simulink model "TV_2017old"  (R2016a)
settings: Solver=FixedStepAuto  StartTime=0.0  StopTime=inf  FixedStep=0.001  RelTol=1e-3
PreLoadFcn:
  | TV_2017_parameters
values from neighbouring files (symbols this model uses):
  battery_voltage = single(530)    [HIL_parameters.m]    (also in HIL_parameters_2018.m; TV_2017_parameters.m; TV_2017_parameters_VD.m)
  car_params = Simulink_Car_params    [HIL_parameters.m]    (also in HIL_parameters_2018.m; TV_2017_parameters.m; TV_2017_parameters_VD.m)
  i_Diff = 16    [HIL_parameters.m]    (also in HIL_parameters_2018.m; TV_2017_parameters.m)
  Kp = 1    [HIL_parameters.m]    (also in HIL_parameters_2018.m; TV_2017_parameters.m; TV_2017_parameters_VD.m)
  motor_data = struct    [HIL_parameters.m]    (also in HIL_parameters_2018.m; TV_2017_parameters.m)
  powerLimitControl = Simulink_el    [HIL_parameters.m]    (also in HIL_parameters_2018.m; TV_2017_parameters.m; TV_2017_parameters_VD.m)
  settings = Simulink_Settings    [HIL_parameters.m]    (also in HIL_parameters_2018.m; TV_2017_parameters.m; TV_2017_parameters_VD.m)
  SpdC_BCC = 0    [HIL_parameters.m]    (also in HIL_parameters_2018.m; TV_2017_parameters.m; TV_2017_parameters_VD.m)
  Speed_Neg_sat = -21    [HIL_parameters.m]    (also in HIL_parameters_2018.m; TV_2017_parameters.m; TV_2017_parameters_VD.m)
  Speed_Pos_sat = 21    [HIL_parameters.m]    (also in HIL_parameters_2018.m; TV_2017_parameters.m; TV_2017_parameters_VD.m)
  SteeringAngleFL = [-23.80 -22.65 -21.50 -20.34 -19.18 -18.03 -16.86 -15.70 -14.53 -13.35 -12.18 -10.99 -9.80 -8.61 -7.40 -6.19 -4.97 -3.75 -2.51 -1.26 0 1.27 2.56 3.85 5.17 6.50 7.84 9.21 10.59 12.00 13.42 14.88 16.36 17.87 19.41 20.99 22.61 24.26 25.97 27.73 29.54]    [CarSetupAnalysis2018.m]    (also in HIL_parameters_2018.m; TV_2017_parameters.m; TV_2017_parameters_VD.m = [-24.129 -22.950 -21.772 -20.593 -19.413 -18.232 -17.050 -15)
  SteeringAngleFR = [-29.54 -27.73 -25.97 -24.26 -22.61 -20.99 -19.41 -17.87 -16.36 -14.88 -13.42 -12.00 -10.59 -9.21 -7.84 -6.50 -5.17 -3.85 -2.56 -1.27 0 1.26 2.51 3.75 4.97 6.19 7.40 8.61 9.80 10.99 12.18 13.35 14.53 15.70 16.86 18.03 19.18 20.34 21.50 22.65 23.80]    [CarSetupAnalysis2018.m]    (also in HIL_parameters_2018.m; TV_2017_parameters.m; TV_2017_parameters_VD.m = [-29.3050 -27.5340 -25.8140 -24.1410 -22.5110 -20.9180 -19.3)
  SteeringWhAngle = [-105 -99.75 -94.5 -89.25 -84 -78.75 -73.5 -68.25 -63 -57.75 -52.5 -47.25 -42 -36.75 -31.5 -26.25 -21.0 -15.75 -10.5 -5.25 0.0 5.25 10.50 15.75 21.00 26.25 31.50 36.75 42.00 47.25 52.50 57.75  63.00 68.25 73.50 78.75 84.00 89.25 94.50 99.75 105.00]    [TV_2017_parameters_VD.m]
  Tn_n = 0    [HIL_parameters.m]    (also in HIL_parameters_2018.m; TV_2017_parameters.m; TV_2017_parameters_VD.m)
  tractionControl = Simulink_tc    [HIL_parameters.m]    (also in HIL_parameters_2018.m; IterativeTractionControlTuning.m; TV_2017_parameters.m; TV_2017_parameters_VD.m)
  yawRateControl = Simulink_yawRate    [HIL_parameters.m]    (also in HIL_parameters_2018.m; TV_2017_parameters.m; TV_2017_parameters_VD.m)
undefined symbols (not defined in the file or in its folder): DiscIntNeverNeededParam, magnitude, speedEstimation, TC_Decr_Gas, TC_Derivative, TC_Incr_Gas, TC_On, TC_Relay_Off, TC_Relay_On
libraries: CarMaker4SL x274, simulink_extras x45, simulink x37, dspfdesign x2
(part 11 of 14)

== matlab function TV_2017old/CarMaker/Control_System /TA 2017/TorqueAllocation ==
  data: Mz_ref input; Ti_lim output Bus: Ti_lim; T_req input; states input; maxMotorTorque input; friction_limit_torques input; settings parameter; car_params parameter; pow_red output; yawRateControl parameter; powerLimitControl parameter; Mz_error output; Mz_allocated output; overiterate output
function [Ti_lim, pow_red,Mz_error, Mz_allocated,overiterate] = torqueAllocation(Mz_ref, T_req, states, maxMotorTorque, friction_limit_torques, settings, car_params, yawRateControl, powerLimitControl)
saturated_constraints = int8([0 0 0 0]);
Mz_error = single(0);
Mz_allocated = single(0);
pow_red = int8([0 0 0 0]);
overiterate = int8(0);




switch settings.TV_Method
    case 1 
        [Ti_lim, pow_red,Mz_error, Mz_allocated] = TA_17(Mz_ref, T_req, states, maxMotorTorque,friction_limit_torques, settings, car_params, yawRateControl, powerLimitControl);    
    case 2
        [Ti_lim,Ti_max,Mz_error, Mz_allocated] = TA_16(T_req,states,maxMotorTorque,settings, car_params, Mz_ref,yawRateControl);   
    case 3
        [Ti_lim,Ti_max,Mz_error, Mz_allocated] = TA_16(T_req,states,maxMotorTorque,settings, car_params, Mz_ref,yawRateControl);
    case 4
        [Ti_lim,Ti_max,Mz_error, Mz_allocated] = TA_16(T_req,states,maxMotorTorque,settings, car_params, Mz_ref,yawRateControl);
    otherwise
        Ti_lim_struct.FL =  single(0); Ti_lim_struct.FR =  single(0); Ti_lim_struct.RL = single(0); Ti_lim_struct.RR =  single(0);
        Ti_lim = Ti_lim_struct;
      
end





end
%{
function [Ti_lim, saturated_constraints,Mz_error, Mz_allocated] = TA_17(Mz_ref, T_req, states, maxMotorTorque,friction_limit_torques, settings, car_params, yawRateControl, powerLimitControl)

%-----variables
error = 0;
pow_red = 0;
max_matrix_dimention = 17;
Ti_max = [0 0 0 0];
Mz_allocated = single(0);
saturated_constraints = int8([0 0 0 0]);
pow_lim_en = powerLimitControl.enable;

% ------- STATES -------------
r = states.r;
negative_torque_limit = yawRateControl.negative_torque_limit;

%---------- PARAMETERS -------
TV_method = settings.TV_Method;
% motor torque limits  
max_motor_torque = single(settings.max_motor_torque);  % absolute limit
negative_torque_limit = yawRateControl.negative_torque_limit;   % max negative DYC torque while accelerating
max_motor_brake_torque = settings.max_motor_brake_torque;   % max brake torque (decelerating)

mu = settings.mu;
lf = car_params.l_f;
lr = car_params.l_r;
tf = car_params.t_f;
tr = car_params.t_r;
arm_f = sqrt(tf^2 + lf^2);
GR = car_params.GR;
r_eff = car_params.r_eff;
R = [r_eff, r_eff, r_eff, r_eff]; % todo -> account for load
delta = states.wheel_angle;
delta_FL = delta;   % fix for later  ->individual steer angles
delta_FR = delta;
T_abs = abs(T_req); 
Mz_ref_scaled = single(Mz_ref * single(yawRateControl.enable));
Mz_min = -yawRateControl.max_moment;
Mz_max = yawRateControl.max_moment;
pow_lim         = powerLimitControl.positive_power_limit; %= single(75000); % Positive effect limit
neg_pow_lim     = powerLimitControl.negative_power_limit;
V_x = states.V_x;



rads_FL = max(10,abs(states.RPM_FL))*2*pi/60  ;
rads_FR = max(10,abs(states.RPM_FR))*2*pi/60  ;
rads_RL = max(10,abs(states.RPM_RL))*2*pi/60  ;
rads_RR = max(10,abs(states.RPM_RR))*2*pi/60  ;

RPM_FL = single(max(500,states.RPM_FL));
RPM_FR = single(max(500,states.RPM_FR));
RPM_RL = single(max(500,states.RPM_RL));
RPM_RR = single(max(500,states.RPM_RR));

mmt_FL = min(max_motor_torque, max(0.1, maxMotorTorque.mmt_FL));  % indivudual max torques
mmt_FR = min(max_motor_torque, max(0.1, maxMotorTorque.mmt_FR)); 
mmt_RL = min(max_motor_torque, max(0.1, maxMotorTorque.mmt_RL)); 
mmt_RR = min(max_motor_torque, max(0.1, maxMotorTorque.mmt_RR));

minmt_FL = min([mmt_FL max_motor_brake_torque]);  % indivudual min torques
minmt_FR = min([mmt_FR max_motor_brake_torque]);
minmt_RL = min([mmt_RL max_motor_brake_torque]);
minmt_RR = min([mmt_RR max_motor_brake_torque]);

max_neg_corr_torque_FL = min([minmt_FL negative_torque_limit]);  % indivudual min torques as corrective moment during acceleration
max_neg_corr_torque_FR = min([minmt_FR negative_torque_limit]); 
max_neg_corr_torque_RL = min([minmt_RL negative_torque_limit]);
max_neg_corr_torque_RR = min([minmt_RR negative_torque_limit]);

%***************************************************


%***************************************************
motor_eff_table = single(100*reshape([0.6437000036239624,0.5799999833106995,0.44999998807907104,0.3499999940395355,0.28999999165534973,0.23999999463558197,0.20000000298023224,0.17000000178813934,0.14000000059604645,0.12999999523162842,0.10999999940395355,0.7099999785423279,0.699999988079071,0.6100000143051148,0.5099999904632568,0.4399999976158142,0.3799999952316284,0.33000001311302185,0.28999999165534973,0.25,0.2199999988079071,0.20000000298023224,0.7300000190734863,0.7699999809265137,0.7300000190734863,0.6700000166893005,0.6100000143051148,0.550000011920929,0.5,0.44999998807907104,0.4000000059604645,0.36000001430511475,0.33000001311302185,0.7400000095367432,0.800000011920929,0.7900000214576721,0.7400000095367432,0.6899999976158142,0.6399999856948853,0.5899999737739563,0.5400000214576721,0.5,0.46000000834465027,0.41999998688697815,0.75,0.8199999928474426,0.8199999928474426,0.7799999713897705,0.7400000095367432,0.699999988079071,0.6600000262260437,0.6100000143051148,0.5699999928474426,0.5299999713897705,0.49000000953674316,0.7599999904632568,0.8399999737739563,0.8500000238418579,0.8299999833106995,0.800000011920929,0.7699999809265137,0.7400000095367432,0.699999988079071,0.6600000262260437,0.6200000047683716,0.5899999737739563,0.7699999809265137,0.8500000238418579,0.8799999952316284,0.8700000047683716,0.8600000143051148,0.8399999737739563,0.8100000023841858,0.7799999713897705,0.7599999904632568,0.7200000286102295,0.699999988079071,0.7699999809265137,0.8500000238418579,0.8899999856948853,0.8799999952316284,0.8700000047683716,0.8500000238418579,0.8299999833106995,0.8100000023841858,0.7799999713897705,0.7599999904632568,0.7300000190734863,0.7699999809265137,0.8600000143051148,0.8999999761581421,0.8999999761581421,0.8899999856948853,0.8700000047683716,0.8500000238418579,0.8299999833106995,0.8100000023841858,0.7900000214576721,0.6700000166893005,0.7799999713897705,0.8600000143051148,0.8999999761581421,0.9100000262260437,0.8999999761581421,0.8899999856948853,0.8700000047683716,0.8600000143051148,0.8299999833106995,0.7699999809265137,0.699999988079071],11,10));
eff_torque_break = single([1.3,2.7,5.4,7.9,10.4,12.5,14.4,16.0,17.4,18.5,25]);
eff_rpm_break = single([500,1000,2000,3000,4000,6000,10000,12000,15000,21000]);
%min_RPM  = min([RPM_FL RPM_FR RPM_RL RPM_RR]);
min_RPM =max(500, V_x* GR * 60 * 1/(pi*2*r_eff) );%using speed to avoid oscillations
min_rads = min([rads_FL,rads_FR,rads_RL,rads_RR]);
max_rads = max([rads_FL,rads_FR,rads_RL,rads_RR]);
%eta_min_RPM = 100/interp2(eff_rpm_break,eff_torque_break,motor_eff_table,min_RPM,max(1.3,x_0(1)));
%***************************************************
fric_lim = friction_limit_torques;
fric_lim = [max(fric_lim(1),1)  max(fric_lim(2),1)  max(fric_lim(3),1)  max(fric_lim(4),1)];
%***************************************************
M_T_FL =     GR/R(1) *  -sin(  atan(tf/lf)  -  delta_FL)  *arm_f;
M_T_FR =     GR/R(2) *   sin(  atan(tf/lf)  +  delta_FR)  *arm_f;
M_T_RL =     GR/R(3) *  -tr;
M_T_RR =     GR/R(4) *   tr;

%***************************************************
sign_reward = 0.5; 
corrective_weight =10^-2;       %10^2;%10^-1;% 10^1;%  G_1
friction_weight   =1;           %10^0;%10^3;      %  G_2
sign_weight =0;                 % friction_weight; % G_3
identity_weight = 0;            %     10            G_4
avoid_neg_num_weight = 0;       % c_4

G_1       = 2*[M_T_FL^2         ,          M_T_FL *M_T_FR   ,       M_T_FL*M_T_RL   ,        M_T_FL*M_T_RR    ;
               M_T_FR * M_T_FL    ,         M_T_FR^2        ,       M_T_FR*M_T_RL   ,        M_T_FR*M_T_RR    ;
               M_T_RL * M_T_FL    ,        M_T_RL*M_T_FR      ,       M_T_RL^2      ,        M_T_RL*M_T_RR    ;
               M_T_RR * M_T_FL    ,        M_T_RR*M_T_FR      ,      M_T_RR* M_T_RL   ,           M_T_RR^2  ];

c_1       = [M_T_FL  , M_T_FR  , M_T_RL  ,  M_T_RR    ]'*(-2)*Mz_ref_scaled;  % **-** this is reformulated after adjusting Mz              
           
G_2  =[        2/fric_lim(1)^2,    0,               0,                  0;
                  0,          2/fric_lim(2)^2,      0,                  0;
                  0,               0,           2/fric_lim(3)^2,        0;
                  0,               0,               0,          2/fric_lim(4)^2];
                
G_3  =eye(4)-[    0,             0,               1,           0;
                  0,             0,               0,           1;
                  1,             0,               0,           0,    ;
                  0,             1,               0,           0]*sign_reward;

G_4 = eye(4);             

c_4 = -[1 1 1 1]'; % n/a..

G = G_1*corrective_weight + friction_weight*G_2+ eye(4)*1/100; %  + sign_weight*G_3 + identity_weight * G_4;  % G_1 should dominate- G_2 should result in values {0,10} in the range where G_1 is minimized
c = c_1*corrective_weight; %  + c_4*avoid_neg_num_weight;   

A_eq   =  single([ 1   1   1   1 ]);
b_eq   =  T_req  ;
eta = 1;

A      =     single(-[min_rads(1),  min_rads(2)  ,   min_rads(3),   min_rads(4)    ;
                         1    ,       0    ,       0    ,        0      ;
                         0    ,       1    ,       0    ,        0      ;
                         0    ,       0    ,       1    ,        0      ;
                         0    ,       0    ,       0    ,        1      ;
                        -1    ,       0    ,       0    ,        0      ;
                         0    ,      -1    ,       0    ,        0      ;
                         0    ,       0    ,      -1    ,        0      ;
                         0    ,       0    ,       0    ,       -1      ]);

% A_2 without pow_lim scale befor optimization instead ... for now     ...              
A_2 = single(-[          1    ,       0    ,       0    ,        0      ;
                         0    ,       1    ,       0    ,        0      ;
                         0    ,       0    ,       1    ,        0      ;
                         0    ,       0    ,       0    ,        1      ;
                        -1    ,       0    ,       0    ,        0      ;
                         0    ,      -1    ,       0    ,        0      ;
                         0    ,       0    ,      -1    ,        0      ;
                         0    ,       0    ,       0    ,       -1      ]);

b    =  -[100000 ,  mmt_FL  ,    mmt_FR  ,    mmt_RL  ,     mmt_RR    , minmt_FL  ,  minmt_FR  ,  minmt_RL  ,   minmt_RR ]'; % pow_lim at pos 1
b_dec    =  -[       0  ,        0   ,       0    ,        0      , minmt_FL  ,  minmt_FR  ,  minmt_RL  ,   minmt_RR ]';
b_acc    =  -[  mmt_FL  ,    mmt_FR  ,    mmt_RL  ,     mmt_RR    , max_neg_corr_torque_FL  ,  max_neg_corr_torque_FR  ,  max_neg_corr_torque_RL  ,   max_neg_corr_torque_RR ]';

% ------------------- POWLIM not done .... edit: is done for now? -> compensate for efficiency later?`-------------------

%Determine feasible startingpoint  / e.v  scale problem
%function [b_eq, x_o]  = determine_feasible_startingpoint(A,b,b_eq,pow_lim,T)
%Limit M_z to avoid allocations with different signedness on one vehicle
%side 


% increase Mz gradually (multiply by 0-1) from V_x = 0 | throtle = 0 up to
% a certain threshold  0  _/  1
V_x_1 = 0.5;   % 1.3 kmh
V_x_2 = 1.5;    %  4ish kmh

if (0<V_x) && (V_x < V_x_1) 
    Mz_Vx_scale = single(0);
elseif (0<V_x) && (V_x < V_x_2)
    Mz_Vx_scale = single(   1   * ( (V_x  -  V_x_1)  / (V_x_2 - V_x_1) ) );
elseif (0<V_x) && (V_x < 150) 
    Mz_Vx_scale = single(1);
else 
    Mz_Vx_scale = single(0);
end

T_a = 0;
T_b = 15; % 1
if T_abs < T_a
    Mz_apps_scale = single(0);
elseif T_abs < T_b
    Mz_apps_scale = single(1  * (    ( T_abs - T_a ) / (T_b - T_a)      ));
else
    Mz_apps_scale = single(1);
end




%-------------------------------------DEBUG-start
if T_req > ( mmt_FL + mmt_FR + mmt_RL +  mmt_RR)
    thisisbreakpoint = 1;
end
%_____________________________________DEBUG-end
%-----------find feasible startingpoint
%--start by finding torque scalingfactor
if b_eq > 0
    b_eq = (min(T_req,( mmt_FL + mmt_FR + mmt_RL +  mmt_RR) )-0.0001);
    beta = b_eq /( mmt_FL + mmt_FR + mmt_RL +  mmt_RR);
elseif b_eq < 0 
    b_eq = (max(T_req,-( minmt_FL + minmt_FR + minmt_RL +  minmt_RR) )+0.0001);
    beta = b_eq /( minmt_FL + minmt_FR + minmt_RL  +  minmt_RR); 
else
    beta = single(0);
end


if (beta < 1)&&(beta > 0.001) % a feasible startingpoint exists (considering b(2:end))
    
    x_0 = beta * [ mmt_FL  ,    mmt_FR  ,    mmt_RL  ,     mmt_RR  ]';
    eta_min_RPM = 85/interp2(eff_rpm_break,eff_torque_break,motor_eff_table,min_RPM,max(1.3,(b_eq/4)));
    %A(1,:) = -[min_rads*eta_min_RPM ,   min_rads*eta_min_RPM ,   min_rads*eta_min_RPM ,    min_rads*eta_min_RPM];
    power = -A(1,:)*x_0*eta_min_RPM;
    
    if power>pow_lim    % ensure feasible startingpoint with regards to powerlimit A(1;:)
        b_eq = b_eq * (pow_lim/power)* 0.99;
        beta_2 = b_eq /( mmt_FL + mmt_FR + mmt_RL + mmt_RR);
        x_0 =   beta_2*[ mmt_FL , mmt_FR , mmt_RL , mmt_RR ]';

    else
        %disp('less than pow_lim')
    end
    
    %_________limit Mz to avoid unequal signedness on one side
    
    if b_eq>(mmt_FL+mmt_RL)
        Mz_min = mmt_FL * M_T_FL +  mmt_RL * M_T_RL + min(M_T_FR , M_T_RR)*(b_eq - mmt_FL- mmt_RL) +10; %-10 to be safe
    end
    if b_eq>(mmt_FR+mmt_RR)
        Mz_max = mmt_FR * M_T_FR + mmt_RR * M_T_RR + max( M_T_FL , M_T_RL)*(b_eq - mmt_FR-mmt_RR) -10 ;
    end
    Mz_ref_scaled = min([Mz_ref_scaled,Mz_max,yawRateControl.max_moment]);
    Mz_ref_scaled = max([Mz_ref_scaled,Mz_min,-yawRateControl.max_moment]);
    
    if (Mz_ref_scaled < Mz_ref-1)
        debugbreakpoint = 1;
    end    
    c_1       = [M_T_FL  , M_T_FR  , M_T_RL  ,  M_T_RR    ]'*-2* Mz_ref_scaled * Mz_Vx_scale * Mz_apps_scale;
    c = c_1*corrective_weight;
    
    %_________limit Mz to avoid unequal signedness on one side ---- end
    
    x = active_set(G,c,A_2,b_acc,A_eq,b_eq,x_0);

    
elseif (beta >= 1) % a feasible startingpoint does not exist (considering b(2:end)) // this don happen with new b_eq scaling
    x_0 = [ mmt_FL  ,    mmt_FR  ,    mmt_RL  ,     mmt_RR  ]'; 
    eta_min_RPM = 100/interp2(eff_rpm_break,eff_torque_break,motor_eff_table,min_RPM,max(1.3,(b_eq/4)));
    %A(1,:) = -[min_rads*eta_min_RPM ,   min_rads*eta_min_RPM ,   min_rads*eta_min_RPM ,    min_rads*eta_min_RPM];
    power = -A(1,:)*x_0;
    if power>pow_lim
        b_eq = T_req * (pow_lim/power)* 0.99;
%         x_0 = x_0*(pow_lim/power)* 0.99;   % added 0.99 factor to "loosen up" the problem
        pow_red = 1;
        beta_2 = b_eq /( mmt_FL + mmt_FR + mmt_RL + mmt_RR);
        x_0 = beta_2 *  [ mmt_FL  ,    mmt_FR  ,    mmt_RL  ,     mmt_RR  ]';
        
        %disp('active openLoop pow_lim')
    else
        %disp('less than pow_lim')
    end
    
    
    %_________limit Mz to avoid unequal signedness on one side
    
    if b_eq>(mmt_FL+mmt_RL)
        Mz_min = mmt_FL * M_T_FL +  mmt_RL * M_T_RL + min(M_T_FR , M_T_RR)*(b_eq - mmt_FL- mmt_RL) +10; %-10 to be safe
    end
    if b_eq>(mmt_FR+mmt_RR)
        Mz_max = mmt_FR * M_T_FR + mmt_RR * M_T_RR + max( M_T_FL , M_T_RL)*(b_eq - mmt_FR-mmt_RR) -10 ;
    end
    Mz_ref_scaled = min([Mz_ref_scaled,Mz_max,yawRateControl.max_moment]);
    Mz_ref_scaled = max([Mz_ref_scaled,Mz_min,-yawRateControl.max_moment]);
    
    c_1       = [M_T_FL  , M_T_FR  , M_T_RL  ,  M_T_RR    ]'*-2* Mz_ref_scaled * Mz_Vx_scale * Mz_apps_scale;
    c = c_1*corrective_weight;
    %_________limit Mz to avoid unequal signedness on one side ---- end
    x = active_set(G,c,A_2,b_acc,A_eq,b_eq,x_0); 

    
elseif (beta > -1)&&(beta < -0.001) % a feasible startingpoint exists (considering b(2:end))
    
    
    x_0 =  beta*[ minmt_FL  ,    minmt_FR  ,    minmt_RL  ,     minmt_RR  ]'; 
    eta_min_RPM = 100/interp2(eff_rpm_break,eff_torque_break,motor_eff_table,min_RPM,max(1.3,(b_eq/4)));
    %A(1,:) = -[min_rads*eta_min_RPM ,   min_rads*eta_min_RPM ,   min_rads*eta_min_RPM ,    min_rads*eta_min_RPM];
    power =  [max_rads max_rads max_rads max_rads]  *x_0;
    if abs(power)>abs(neg_pow_lim)
        b_eq = b_eq * (abs(neg_pow_lim)/abs(power))* 0.99;
        %x_0 = x_0*(abs(pow_lim)/abs(power))* 0.99;   % added 0.99 factor to "loosen up" the problem
        pow_red = 1;
        
        
        beta_2 = abs( b_eq /( minmt_FL + minmt_FR + minmt_RL + minmt_RR) ) ;
        x_0 = -beta_2 *  [ minmt_FL  ,    minmt_FR  ,    minmt_RL  ,     minmt_RR  ]';
        %disp('active openLoop pow_lim')
    else
        %disp('less than pow_lim')
    end
   
    Mz_min = (-minmt_FR * M_T_FR) +  (-minmt_RR * M_T_RR) ; %-10 to be safe
    Mz_max = (-minmt_FL * M_T_FL) +  (-minmt_RL * M_T_RL) ;
    
    Mz_ref_scaled = min([Mz_ref_scaled,Mz_max,yawRateControl.max_moment]);
    Mz_ref_scaled = max([Mz_ref_scaled,Mz_min,-yawRateControl.max_moment]);
    
    c_1       = [M_T_FL  , M_T_FR  , M_T_RL  ,  M_T_RR    ]'*-2* Mz_ref_scaled * Mz_Vx_scale ;
    c = c_1*corrective_weight;
    
    x = active_set(G,c,A_2,b_dec,A_eq,b_eq,x_0); 
    if max(x)> 0.5
        hmmm = 1;
    end
elseif (beta <= -1) % a feasible startingpoint does not exist (considering b(2:end)) // this dont happen with new b_eq scaling
    x_0 = -[minmt_FL  ,  minmt_FR  ,  minmt_RL  ,   minmt_RR ]'; 
    %FIX negative powerlimiting
    x = x_0;
else
    x = zeros(4,1,'single'); %default case, should not happen
end


if x(4)>7 %% debug statement
    stophere = 1;
end


Mz_ref_scaled;
% add constraints active based on lambda
Mz_allocated = [M_T_FL  , M_T_FR  , M_T_RL  ,  M_T_RR  ]* x;
Mz_error = Mz_ref - Mz_allocated;
Ti_lim_struct    = struct;
Ti_lim_struct.FL = x(1); Ti_lim_struct.FR = x(2); Ti_lim_struct.RL = x(3); Ti_lim_struct.RR = x(4);
Ti_lim = Ti_lim_struct;
x'*G*x+x'*c;
end

%}


function [Ti_lim, saturated_constraints,Mz_error, Mz_allocated] = TA_17(Mz_ref, T_req, states, maxMotorTorque,friction_limit_torques, settings, car_params, yawRateControl, powerLimitControl)
%-----variables
error = 0;
pow_red = 0;
max_matrix_dimention = 17;
Ti_max = [0 0 0 0];
Mz_allocated = single(0);
saturated_constraints = int8([0 0 0 0]);
pow_lim_en = powerLimitControl.enable;

% ------- STATES -------------
r = states.r;
negative_torque_limit = yawRateControl.negative_torque_limit;

%---------- PARAMETERS -------
TV_method = settings.TV_Method;
mmt = single(settings.max_motor_torque);
mu = settings.mu;
lf = car_params.l_f;
lr = car_params.l_r;
tf = car_params.t_f;
tr = car_params.t_r;
arm_f = sqrt(tf^2 + lf^2);
GR = car_params.GR;
r_eff = car_params.r_eff;
R = [r_eff, r_eff, r_eff, r_eff]; % todo -> account for load
delta = states.wheel_angle;
delta_FL = delta;   % fix for later  ->individual steer angles
delta_FR = delta;
T_abs = abs(T_req); 
Mz_ref_scaled = single(Mz_ref * single(yawRateControl.enable));
pow_lim         = powerLimitControl.positive_power_limit; %= single(75000); % Positive effect limit
neg_pow_lim     = powerLimitControl.negative_power_limit;


if states.V_x < 1
    Mz_ref_scaled = single(0);
elseif states.V_x < 3
    Mz_ref_scaled = single(Mz_ref_scaled/(states.V_x/5));
else
    Mz_ref_scaled = Mz_ref_scaled;
end




rads_FL = max(10,abs(states.RPM_FL))*2*pi/60  ;
rads_FR = max(10,abs(states.RPM_FR))*2*pi/60  ;
rads_RL = max(10,abs(states.RPM_RL))*2*pi/60  ;
rads_RR = max(10,abs(states.RPM_RR))*2*pi/60  ;

RPM_FL = single(max(500,states.RPM_FL));
RPM_FR = single(max(500,states.RPM_FR));
RPM_RL = single(max(500,states.RPM_RL));
RPM_RR = single(max(500,states.RPM_RR));

mmt_FL = min(mmt, max(0.1, maxMotorTorque.mmt_FL));  % fix ned limit later
mmt_FR = min(mmt, max(0.1, maxMotorTorque.mmt_FR)); 
mmt_RL = min(mmt, max(0.1, maxMotorTorque.mmt_RL)); 
mmt_RR = min(mmt, max(0.1, maxMotorTorque.mmt_RR)); 
minmt_FL = min([mmt_FL settings.max_motor_brake_torque]);
minmt_FR = min([mmt_FR settings.max_motor_brake_torque]);
minmt_RL = min([mmt_RL settings.max_motor_brake_torque]);
minmt_RR = min([mmt_RR settings.max_motor_brake_torque]);
%***************************************************
motor_eff_table = single(100*reshape([0.6437000036239624,0.5799999833106995,0.44999998807907104,0.3499999940395355,0.28999999165534973,0.23999999463558197,0.20000000298023224,0.17000000178813934,0.14000000059604645,0.12999999523162842,0.10999999940395355,0.7099999785423279,0.699999988079071,0.6100000143051148,0.5099999904632568,0.4399999976158142,0.3799999952316284,0.33000001311302185,0.28999999165534973,0.25,0.2199999988079071,0.20000000298023224,0.7300000190734863,0.7699999809265137,0.7300000190734863,0.6700000166893005,0.6100000143051148,0.550000011920929,0.5,0.44999998807907104,0.4000000059604645,0.36000001430511475,0.33000001311302185,0.7400000095367432,0.800000011920929,0.7900000214576721,0.7400000095367432,0.6899999976158142,0.6399999856948853,0.5899999737739563,0.5400000214576721,0.5,0.46000000834465027,0.41999998688697815,0.75,0.8199999928474426,0.8199999928474426,0.7799999713897705,0.7400000095367432,0.699999988079071,0.6600000262260437,0.6100000143051148,0.5699999928474426,0.5299999713897705,0.49000000953674316,0.7599999904632568,0.8399999737739563,0.8500000238418579,0.8299999833106995,0.800000011920929,0.7699999809265137,0.7400000095367432,0.699999988079071,0.6600000262260437,0.6200000047683716,0.5899999737739563,0.7699999809265137,0.8500000238418579,0.8799999952316284,0.8700000047683716,0.8600000143051148,0.8399999737739563,0.8100000023841858,0.7799999713897705,0.7599999904632568,0.7200000286102295,0.699999988079071,0.7699999809265137,0.8500000238418579,0.8899999856948853,0.8799999952316284,0.8700000047683716,0.8500000238418579,0.8299999833106995,0.8100000023841858,0.7799999713897705,0.7599999904632568,0.7300000190734863,0.7699999809265137,0.8600000143051148,0.8999999761581421,0.8999999761581421,0.8899999856948853,0.8700000047683716,0.8500000238418579,0.8299999833106995,0.8100000023841858,0.7900000214576721,0.6700000166893005,0.7799999713897705,0.8600000143051148,0.8999999761581421,0.9100000262260437,0.8999999761581421,0.8899999856948853,0.8700000047683716,0.8600000143051148,0.8299999833106995,0.7699999809265137,0.699999988079071],11,10));
eff_torque_break = single([1.3,2.7,5.4,7.9,10.4,12.5,14.4,16.0,17.4,18.5,25]);
eff_rpm_break = single([500,1000,2000,3000,4000,6000,10000,12000,15000,21000]);
%***************************************************
fric_lim = friction_limit_torques;
%***************************************************
M_T_FL =     GR/R(1) *  -sin(  atan(tf/lf)  -  delta_FL)  *arm_f;
M_T_FR =     GR/R(2) *   sin(  atan(tf/lf)  +  delta_FR)  *arm_f;
M_T_RL =     GR/R(3) *  -tr;
M_T_RR =     GR/R(4) *   tr;
%***************************************************

G_1       = 2*[ M_T_FL^2          ,          M_T_FL *M_T_FR   ,       M_T_FL*M_T_RL   ,        M_T_FL*M_T_RR    ;
               M_T_FR * M_T_FL    ,           M_T_FR^2        ,       M_T_FR*M_T_RL   ,        M_T_FR*M_T_RR    ;
               M_T_RL * M_T_FL    ,        M_T_RL*M_T_FR      ,         M_T_RL^2      ,        M_T_RL*M_T_RR    ;
               M_T_RR * M_T_FL    ,        M_T_RR*M_T_FR      ,      M_T_RR* M_T_RL   ,              M_T_RR^2  ];

c_1       = [M_T_FL  , M_T_FR  , M_T_RL  ,  M_T_RR    ]'*-2*Mz_ref_scaled;                
           
L_CT = 1;%left side cross term. To ensure that the torques have the same direction on the left side of the car.
R_CT = 1;%right side cross term. To ensure that the torques have the same direction on the right side of the car.

G_2  =[        2/fric_lim(1)^2,    0,               -L_CT,                  0;
                  0,          2/fric_lim(2)^2,      0,                  -R_CT;
                  -L_CT,               0,           2/fric_lim(3)^2,        0;
                  0,               -R_CT,               0,          2/fric_lim(4)^2];             

G = G_1/100 + 10*G_2;  
c = c_1/100;

A_eq   =  single([ 1   1   1   1 ]);
b_eq   =  T_req ;

A      =     single(-[rads_FL ,   rads_FR ,   rads_RL ,    rads_RR      ;
                         1    ,       0    ,       0    ,        0      ;
                         0    ,       1    ,       0    ,        0      ;
                         0    ,       0    ,       1    ,        0      ;
                         0    ,       0    ,       0    ,        1      ;
                        -1    ,       0    ,       0    ,        0      ;
                         0    ,      -1    ,       0    ,        0      ;
                         0    ,       0    ,      -1    ,        0      ;
                         0    ,       0    ,       0    ,       -1      ]);

b    =  -[pow_lim ,  mmt_FL  ,    mmt_FR  ,    mmt_RL  ,     mmt_RR    , minmt_FL  ,  minmt_FR  ,  minmt_RL  ,   minmt_RR ]'; 
% ------------------- POWLIM not done !! is done for now? compensate for efficiency later?`-------------------
%Determine feasible startingpoint  / scale problem
%function [b_eq, x_o]  = determine_feasible_startingpoint(A,b,b_eq,pow_lim,T)
eta_FL = single(1);
eta_FR = single(1);
eta_RL = single(1);
eta_RR = single(1);
%disp('Beta >= 1');

if b_eq > 0.001
    %b_eq = (min(T_req,( mmt_FL + mmt_FR + mmt_RL +  mmt_RR) )-0.0001);
    beta = b_eq /( mmt_FL + mmt_FR + mmt_RL +  mmt_RR);
elseif b_eq < -0.001 
    %b_eq = (max(T_req,-( minmt_FL + minmt_FR + minmt_RL +  minmt_RR) )+0.0001);
    beta = b_eq /( minmt_FL + minmt_FR + minmt_RL  +  minmt_RR); 
else
    beta = single(0);
end

disp (beta);
if (beta < 1)&&(beta >= 0) % a feasible startingpoint exists (considering b(2:end))
   
    x_0 = beta * [ mmt_FL  ,    mmt_FR  ,    mmt_RL  ,     mmt_RR  ]';
    if ~pow_lim_en;
    eta_FL = 100/interp2(eff_rpm_break,eff_torque_break,motor_eff_table,RPM_FL,max(1.3,x_0(1)));
    eta_FR = 100/interp2(eff_rpm_break,eff_torque_break,motor_eff_table,RPM_FR,max(1.3,x_0(2)));
    eta_RL = 100/interp2(eff_rpm_break,eff_torque_break,motor_eff_table,RPM_RL,max(1.3,x_0(3)));
    eta_RR = 100/interp2(eff_rpm_break,eff_torque_break,motor_eff_table,RPM_RR,max(1.3,x_0(4)));
    A(1,:) = -[rads_FL*eta_FL ,   rads_FR*eta_FR ,   rads_RL*eta_RL ,    rads_RR*eta_RR];
    end
    pow = -A(1,:)*x_0;
    if pow>pow_lim    % ensure feasible startingpoint with regards to powerlimit A(1;:)
        b_eq = T_req * 1;%(pow_lim/pow);
        x_0 = x_0*(pow_lim/pow);
        if ~pow_lim_en;
        eta_FL = 100/interp2(eff_rpm_break,eff_torque_break,motor_eff_table,RPM_FL,max(1.3,x_0(1)));
        eta_FR = 100/interp2(eff_rpm_break,eff_torque_break,motor_eff_table,RPM_FR,max(1.3,x_0(2)));
        eta_RL = 100/interp2(eff_rpm_break,eff_torque_break,motor_eff_table,RPM_RL,max(1.3,x_0(3)));
        eta_RR = 100/interp2(eff_rpm_break,eff_torque_break,motor_eff_table,RPM_RR,max(1.3,x_0(4)));
        A(1,:) = -[rads_FL*eta_FL ,   rads_FR*eta_FR ,   rads_RL*eta_RL ,    rads_RR*eta_RR];
        end
    end
    x = active_set(G,c,A,b,A_eq,b_eq,x_0); % All good so far
%    disp(x');
elseif (beta > -1)&&(beta < 0) % a feasible startingpoint exists (considering b(2:end))
    x_0 = beta * [minmt_FL  ,  minmt_FR  ,  minmt_RL  ,   minmt_RR ]';
%     if ~pow_lim_en;
%     eta_FL = 100/interp2(eff_rpm_break,eff_torque_break,motor_eff_table,RPM_FL,max(1.3,x_0(1)));
%     eta_FR = 100/interp2(eff_rpm_break,eff_torque_break,motor_eff_table,RPM_FR,max(1.3,x_0(2)));
%     eta_RL = 100/interp2(eff_rpm_break,eff_torque_break,motor_eff_table,RPM_RL,max(1.3,x_0(3)));
%     eta_RR = 100/interp2(eff_rpm_break,eff_torque_break,motor_eff_table,RPM_RR,max(1.3,x_0(4)));
%     A(1,:) = -[rads_FL*eta_FL ,   rads_FR*eta_FR ,   rads_RL*eta_RL ,    rads_RR*eta_RR];
%     end
%     pow = A(1,:)*x_0;
    x = active_set(G,c,A,b,A_eq,b_eq,x_0); 

elseif (beta >= 1) % a feasible startingpoint does not exist (considering b(2:end))
    
    x_0 = [ mmt_FL  ,    mmt_FR  ,    mmt_RL  ,     mmt_RR  ]'; 
    if ~pow_lim_en;
    eta_FL = 100/interp2(eff_rpm_break,eff_torque_break,motor_eff_table,RPM_FL,max(1.3,x_0(1)));
    eta_FR = 100/interp2(eff_rpm_break,eff_torque_break,motor_eff_table,RPM_FR,max(1.3,x_0(2)));
    eta_RL = 100/interp2(eff_rpm_break,eff_torque_break,motor_eff_table,RPM_RL,max(1.3,x_0(3)));
    eta_RR = 100/interp2(eff_rpm_break,eff_torque_break,motor_eff_table,RPM_RR,max(1.3,x_0(4)));
    end
    A(1,:) = -[rads_FL*eta_FL ,   rads_FR*eta_FR ,   rads_RL*eta_RL ,    rads_RR*eta_RR];
    pow = -A(1,:)*x_0;
    if pow>pow_lim
        b_eq = T_req * (pow_lim/pow);
        x_0 = x_0*(pow_lim/pow);
        pow_red = 1;
    end
    x = x_0;
   %disp('Beta >= 1');
elseif (beta < -1) % a feasible startingpoint does not exist (considering b(2:end))
    x_0 = -[minmt_FL  ,  minmt_FR  ,  minmt_RL  ,   minmt_RR ]'; 
    x = x_0;
   % disp('Beta < -1');
else
    x = zeros(4,1,'single'); %default case, should not happen
   % disp('default case');
end

% add constraints active based on lambda
Mz_allocated = [M_T_FL  , M_T_FR  , M_T_RL  ,  M_T_RR  ]* x;
Mz_error = Mz_ref - Mz_allocated;
Ti_lim_struct    = struct;
Ti_lim_struct.FL = x(1); Ti_lim_struct.FR = x(2); Ti_lim_struct.RL = x(3); Ti_lim_struct.RR = x(4);
Ti_lim = Ti_lim_struct;
end

%Active set method for convex QP  ( pg 472 optreg ) 
function [x,W_i] = active_set(G,c,A,b,A_eq,b_eq,x_0)

%0) Formulate KKT matrix

%1) set w_0 to be a subset of the actiive constraints at x_o

%
W_i = zeros(1,size(A,1),'single'); % W_i lists indexes of A in W, such that W_i has size m
x_k = x_0;
x = single(x_0);


debug_main_iteration = 1;
notdone = 1;
iteration_count = 0;

while notdone
    if iteration_count > 22;
%         disp('iteration-count overflow!')
        overiterate = int8(2);
        notdone = 0;
        x = x_k;
    end
    
   %Solve (16.39 to find pk, Where p_k is the feasible direction
    [p_k, all_lambda_positive] = calc_p_and_eval_lambda(G,  c,  A,  b, A_eq,  b_eq, W_i,  x_k );
    
    
    
    %debug-----------------------------------------------------------
%     iteration_count
%     W_i
%     b_eq
%     x_k
%     p_k
    %     
%     [alpha,violating_indexes] = compute_alpha(A,b,x_k,p_k,W_i);
%     de_bug2 = A*(x_k + alpha*p_k) - b;
%     ansr = max(de_bug2);
%     if ansr < -0.01
%         fail = true;
%     end
%     
%     [p_k, all_lambda_positive] = calc_p_and_eval_lambda(G,  c,  A,  b, A_eq,  b_eq, W_i,  x_k ); 
    %debug________________________________________________
    
    %If p_k == 0 => There are no feasible directions
    disp('============NEW ITERATION============')
    disp ('p_k')
    disp (p_k)
    disp ('W_i')
    disp (W_i)
    disp('Iteration_count')
    disp(iteration_count)
    
    if sum(abs(p_k)) < 0.001   % may cause alg to remove index with empty set...
        if all_lambda_positive;   %Then this is the optimal point
            x = x_k;
            notdone = 0;
            %debug----------------
%             iteration_count
%             W_i
            %debug_____________________
        elseif max(W_i)>0 %This greater than is only to ensure not removing indexes from empty set
            %This section is to find the P, such that we move towards the
            %feasible point
            W_i = exclude_most_negative_lambda_index(G,  c,  A,  b,  A_eq,  b_eq,  x_k , W_i);
            iteration_count = iteration_count + 1;
        else
            x = x_k;
            notdone = 0;
            
        end
    elseif sum(abs(p_k)) ~= 0 %There is a feasible direction which reduces X
        
        [alpha,violating_indexes] = compute_alpha(A,b,x_k,p_k,W_i);
        disp ('Violating_indexes')
        disp (violating_indexes)
        disp ('alpha')
        disp(alpha)
        disp ('x_k')
        disp(x_k)
        disp (' ')
        x_k = x_k + alpha*p_k ; %moving to next basic feasible point, and updating the optimal
       
        if alpha < 1 %indicates blocking constraints, as we where not able to move the entire way towards optimal
%           disp('blocking constraints')
%             disp(alpha)
            %add one of blocking constraints to W_k
            new_index = find(violating_indexes,1); %returns index of first non-0 value
            W_i(new_index) = 1;
            iteration_count = iteration_count + 1;
            
        else
             
            iteration_count = iteration_count + 1;
            
        end
    else
        
        x = x_k;
        iteration_count = 20;      
    end
    %W_i
end

% make it based on lambda
end

function [p_val, all_lambda_positive] =  calc_p_and_eval_lambda(G,  c,  A,  b, A_eq,  b_eq, W_i, x_k )
[W,b_w] = construct_working_set(A,  b, A_eq , b_eq ,  W_i);    
[p, lagrangians] = solve_KKT(G,  c,  W,  b_w,  x_k );
p_val = p;
%all_lambda_positive = sum(sign(lagrangians)) == (sum(W_i)+1);% indicates all values are positivr ( sign(0) returns false, will this cause error on loosely active constraints?  edit:  yes it did ....
if length(lagrangians)==1
    all_lambda_positive = uint8(1);
else
    all_lambda_positive = uint8(0<min(lagrangians(2:end)));
end


% if length(lagrangians)==size(b_eq,1)
%     all_lambda_positive = true;
% else
%     all_lambda_positive = min(lagrangians((length(b_eq)+1):end)) >= 0; % indicates all values are positive       
% end
end

function W_i = exclude_most_negative_lambda_index(G,  c,  A,  b,  A_eq, b_eq,  x_k , W_i)
[W,b_w] = construct_working_set(A,  b, A_eq , b_eq , W_i);   
[~, lagrangians] = solve_KKT(G,  c,  W,  b_w,  x_k );
% identify most negative lagrangian / 1 negative is guarranteed to exist
            low_value = single(0);
            low_index = int8(1);
            for j = (length(b_eq)+1):length(lagrangians)
                if lagrangians(j) <= low_value
                    low_value = lagrangians(j);
                    low_index = int8(j-1);
                else
                    %skip
                end
            end
            k = find(W_i,low_index);
%             if k(low_index) > length(W_i)
%                 r=9;
%             end
            W_i(k(low_index)) = 0;
            %W_i(low_index) = 0; % exclude j from IandW
            % construct new working set
            %[W,b_w] = construct_working_set(A_eq, b_eq, A, W_i, b);
            % got out of range error, tried to access second nonzero
            % element in W_i when there only where one nonzero elemnt (pow lim )
            % EDIT: think this is fix now
end

function [p, lambda_s] = solve_KKT(G,  c,  A,  b,  x_k )  % A is the working set W 
    sol = zeros(4+size(A,1),1,'single');
    %   add error handling here? 
    %   G, A and K needs full rank for K to be invertable
    disp('===========KKT SOVLER===========')
    
    h =  A*x_k   -   b           ;
    g =  c       +   G*x_k       ;
    K = [G             A'        ;
         A        zeros(size(A,1),'single')];
    disp('h')
    disp(h)
    disp('g')
    disp(g)
    disp('k')
    disp(K)
     
    sol      =   K\[g ; h];
    p        =   -sol(1:size(G,1));
    lambda_s =    sol((size(G,1)+1):size(G,1)+size(A,1));
end
%{
% function [alpha,violating_indexes] = compute_alpha(A, b , x_k , p_k ,  W_i) %% this is wrong, observed alpha -368.3450
%     
%     violating_indexes = zeros(1,size(A,1));
%     values = ones(1,size(A,1));
%     debug_values = ones(1,size(A,1));
%     for i =  1:size(A,1) 
%         if ~W_i(i)  &&  (A(i,:)*p_k < 0)
%             val = (b(i) - A(i,:)*x_k)/(A(i,:)*p_k);
%             debug_values(i) = val;
%             if 0<=val && val<=1
%                 values(i) = val;
%                 violating_indexes(i) = 1;
%             end
%         else
%             %skip
%         end
%     end
%     alpha = min([1,values]);
% end
%}
function [alpha,violating_indexes] = compute_alpha(A, b , x_k , p_k ,  W_i) %% this is wrong, observed alpha -368.3450
    lowest_alpha_index = 0;
    violating_indexes = zeros(1,size(A,1));
    lowest_violating_indexes = zeros(1,size(A,1));
    values = ones(1,size(A,1));
    debug_values = ones(1,size(A,1));
    for i =  1:size(A,1) 
        if ~W_i(i)  &&  (A(i,:)*p_k < 0)
            val = (b(i) - A(i,:)*x_k)/(A(i,:)*p_k);
            debug_values(i) = val;
            if 0<=val && val<=1
                values(i) = val;
                violating_indexes(i) = 1;
                if val <= min(values)
                    lowest_alpha_index = i;
                end
            end
        else
            %skip
        end
    end
    if lowest_alpha_index
        violating_indexes(lowest_alpha_index) = 1;
    end
        alpha = min([1,values]);
end

function [W,b_w] = construct_working_set(A , b, A_eq , b_eq  , W_i )
W_ineq = zeros( dim_bound(sum(W_i)) , dim_bound(size(A_eq,2)) , 'single' ); 
b_ineq = zeros( dim_bound(sum(W_i)) , 1 , 'single' );
working_set_iterator = 1;
for u=1:size(A,1)
        if W_i(u)==1
            
            W_ineq(working_set_iterator,:) = A(u,:);
            b_ineq(working_set_iterator,1) = b(u);
            working_set_iterator = working_set_iterator + 1;
        end
end
W = [A_eq ; W_ineq]; 
b_w = [b_eq;b_ineq];
end

function y = dim_bound(n)
assert (n <= 17);
y = n;
end

%---------------------------------TA_16---------------------------------------------------------------------------
function [Ti_lim,Ti_max,Mz_error, Mz_allocated]  = TA_16(T_req,states,maxMotorTorque,settings, car_params, Mz_ref,yawRateControl)
%#codegen

%STATES
r = states.r;
negative_torque_limit = yawRateControl.negative_torque_limit;

%PARAMETERS
%mu = states.mu;
mu = settings.mu;
tf = car_params.t_f*2;
tr = car_params.t_r*2;
GR = car_params.GR;
r_eff = car_params.r_eff;
R = [r_eff; r_eff; r_eff; r_eff]';


Fzi = [max(1,states.Fz_FL) max(1,states.Fz_FR) max(1,states.Fz_RL) max(1,states.Fz_RR)]';
switch settings.TV_Method
    case 1
        % QP ASS 2017
       alfa_r =  (Fzi(3) + Fzi(4)) / (Fzi(1) + Fzi(2) + Fzi(3) + Fzi(4));
    case 2
        % Full allocation 2016
       alfa_r =  (Fzi(3) + Fzi(4)) / (Fzi(1) + Fzi(2) + Fzi(3) + Fzi(4));
       %alfa_r = single(0.5)  test dette for å se om distribusjonen blir
       %lik ev soverestimer friksjonspotensialet
    case 3
        % Static 25 percent to each wheel
        alfa_r = single(0.5);
    case 4
        % Allocation with negative torque, but does not use Fz
        alfa_r = single(0.5); 
    otherwise
        alfa_r = single(0.5);       
end

S = states.wheel_angle;

l1 = car_params.t_f*cos(S);
l2 = car_params.t_f*cos(S);
l3 = car_params.t_r;
l4 = car_params.t_r;
L = [-l1; l2; -l3; l4];



%FIND MAXIMUM ALLOWED MOTOR TORQUE, TIRE/MOTOR
Ti_max          = single(zeros(4,1));
Ti_max_tire     = single(zeros(4,1));

RPM = [states.RPM_FL, states.RPM_FR, states.RPM_RL, states.RPM_RR];
Ti_max_motor = [maxMotorTorque.mmt_FL,maxMotorTorque.mmt_FR,maxMotorTorque.mmt_RL,maxMotorTorque.mmt_RR]; 

%Tire saturation based on mu and Fz
for i=1:4
    Ti_max_tire(i) = Fzi(i)*mu*R(i)/GR;
end

%Find minimum of tire saturation Torque and motor
for i=1:4
    Ti_max(i) = min(Ti_max_tire(i), Ti_max_motor(i));
end
%**********************************************%

T_F = single(zeros(2,1));
T_R = single(zeros(2,1));
sat_F = uint32(0);
sat_R = uint32(0);

if ( T_req >= 0)
    switch settings.TV_Method
        case 1
            % QP ASS 2017
            
        case 2
            % Can also allocate negative torque
            [T_F, sat_F] = allocateTorque(Ti_max(1), Ti_max(2), T_req, R(1), R(2), (1-alfa_r), Mz_ref, GR, tf, negative_torque_limit);
            [T_R, sat_R] = allocateTorque(Ti_max(3), Ti_max(4), T_req, R(3), R(4), alfa_r, Mz_ref, GR, tr ,negative_torque_limit);
        case 3
            % Static 25 percent to each wheel
            T_F = [0.25*T_req; 0.25*T_req];
            T_R = [0.25*T_req; 0.25*T_req];
        case 4
            % Allocation with negative torque, but does not use Fz
            [T_F, sat_F] = allocateTorque(Ti_max_motor(1), Ti_max_motor(2), T_req, R(1), R(2), (1-alfa_r), Mz_ref, GR, tf, negative_torque_limit);
            [T_R, sat_R] = allocateTorque(Ti_max_motor(3), Ti_max_motor(4), T_req, R(3), R(4), alfa_r, Mz_ref, GR, tr ,negative_torque_limit);
    end
            
    if ( (sat_F == 1) && (sat_R == 1) )
        % Nothing more to do
    elseif ( (sat_F == 1) && (sat_R == 0) )     
         if ( T_F(1) < 0) 
            T_remaining = T_req - (T_F(2));
         elseif (T_F(2) < 0) 
             T_remaining = T_req - (T_F(1));
         else
             T_remaining = T_req - (T_F(1) + T_F(2));
         end
         
         if (yawRateControl.enable == 1)
             Mz_remaining = Mz_ref - (-l1*GR*T_F(1)/R(1) + l2*GR*T_F(2)/R(2));
         else
             Mz_remaining = single(0);
         end 
         
        switch settings.TV_Method
            case 1
                % Only positive Torque
                [T_R sat_R] = allocatePositiveTorque(Ti_max(3), Ti_max(4), T_remaining, R(3), R(4), 1 , Mz_remaining, GR, tr);
            case 2
                % Can also allocate negative torque
                [T_R sat_R] = allocateTorque(Ti_max(3), Ti_max(4), T_remaining, R(3), R(4), 1 , Mz_remaining, GR, tr,negative_torque_limit);
            case 4
                [T_R sat_R] = allocateTorque(Ti_max_motor(3), Ti_max_motor(4), T_remaining, R(3), R(4), 1 , Mz_remaining, GR, tr,negative_torque_limit);
        end 
    elseif ( (sat_F == 0) && (sat_R == 1) )
         if ( T_R(1) < 0) 
            T_remaining = T_req - (T_R(2));
         elseif (T_R(2) < 0) 
             T_remaining = T_req - (T_R(1));
         else
             T_remaining = T_req - (T_R(1) + T_R(2));
         end        
        % For example rear is saturated, and front can still use more torque
        %T_remaining = T_req - (T_R(1) + T_R(2));
        if (yawRateControl.enable == 1)
             Mz_remaining = Mz_ref - (-l3*GR*T_R(1)/R(3) + l4*GR*T_R(2)/R(4));
        else
             Mz_remaining = single(0);
        end 
        %Mz_remaining = Mz_ref*(1-alfa_r);
        switch settings.TV_Method
            case 1
                % Only positive Torque
                 [T_F sat_F] = allocatePositiveTorque(Ti_max(1), Ti_max(2), T_remaining, R(1), R(2), 1 , Mz_remaining, GR, tf);
            case 2
                % Can also allocate negative torque
                [T_F sat_F] = allocateTorque(Ti_max(1), Ti_max(2), T_remaining, R(1), R(2), 1 , Mz_remaining, GR, tf,negative_torque_limit);
            case 4
                [T_F sat_F] = allocateTorque(Ti_max_motor(1), Ti_max_motor(2), T_remaining, R(1), R(2), 1 , Mz_remaining, GR, tf,negative_torque_limit);
        end      
    else
        %both false
        % Nothing to do here either
    end
else
    %REGENERATIVE BRAKE COMMAND ( T_DRIVER_REQ < 0 )
    switch settings.TV_Method
        case 1
            % Only positive Torque
            [T_F, sat_F] = allocateKersTorque(Ti_max(1), Ti_max(2), T_req, R(1), R(2), (1-alfa_r), Mz_ref, GR, tf);
            [T_R, sat_R] = allocateKersTorque(Ti_max(3), Ti_max(4), T_req, R(3), R(4), alfa_r, Mz_ref, GR, tr);
            
        case 2
            % Can also allocate negative torque
            [T_F, sat_F] = allocateKersTorque(Ti_max(1), Ti_max(2), T_req, R(1), R(2), (1-alfa_r), Mz_ref, GR, tf);
            [T_R, sat_R] = allocateKersTorque(Ti_max(3), Ti_max(4), T_req, R(3), R(4), alfa_r, Mz_ref, GR, tr);
        case 3
            % Static 25 percent to each wheel
            T_F = [0.25*T_req; 0.25*T_req];
            T_R = [0.25*T_req; 0.25*T_req];
        case 4
            % Allocation with negative torque, but does not use Fz
            [T_F, sat_F] = allocateKersTorque(Ti_max_motor(1), Ti_max_motor(2), T_req, R(1), R(2), (1-alfa_r), Mz_ref, GR, tf);
            [T_R, sat_R] = allocateKersTorque(Ti_max_motor(3), Ti_max_motor(4), T_req, R(3), R(4), alfa_r, Mz_ref, GR, tr);
    end
    if (sat_F == 1 && sat_R == 1)
        %Nothing more to do
        
    elseif (sat_F == 1 && sat_R == 0)
         T_remaining = T_req - (T_F(1) + T_F(2));
         %Disable Mz_remaining if yaw control disabled?
        if (yawRateControl.enable == 1)
             Mz_remaining = Mz_ref - (-l1*GR*T_F(1)/R(1) + l2*GR*T_F(2)/R(2));
        else
             Mz_remaining = single(0);
        end
        switch settings.TV_Method
            case 1
                % Only positive Torque
                [T_R sat_R] = allocateKersTorque(Ti_max(3), Ti_max(4), T_remaining, R(3), R(4), 1 , Mz_remaining, GR, tr);

            case 2
                % Can also allocate negative torque
                [T_R sat_R] = allocateKersTorque(Ti_max(3), Ti_max(4), T_remaining, R(3), R(4), 1 , Mz_remaining, GR, tr);
            case 3
                % Static 25 %
            case 4
                % Allocation with negative torque, but does not use Fz
                [T_R sat_R] = allocateKersTorque(Ti_max_motor(3), Ti_max_motor(4), T_remaining, R(3), R(4), 1 , Mz_remaining, GR, tr);
        end
        
    elseif (sat_F == 0 && sat_R == 1)
        %For example rear is saturated, and front can still use more torque
        T_remaining = T_req - (T_R(1) + T_R(2));
        %Mz_remaining = Mz_ref*(1-alfa_r);
        
        if (yawRateControl.enable == 1)
             Mz_remaining = Mz_ref - (-l3*GR*T_R(1)/R(3) + l4*GR*T_R(2)/R(4));
        else
             Mz_remaining = single(0);
        end
        switch settings.TV_Method
            case 1
                % Only positive Torque
                [T_F sat_F] = allocateKersTorque(Ti_max(1), Ti_max(2), T_remaining, R(1), R(2), 1 , Mz_remaining, GR, tf); 

            case 2
                % Can also allocate negative torque
                [T_F sat_F] = allocateKersTorque(Ti_max(1), Ti_max(2), T_remaining, R(1), R(2), 1 , Mz_remaining, GR, tf); 
            case 3
                % Static 25 %
            case 4
                % Allocation with negative torque, but does not use Fz
                [T_F sat_F] = allocateKersTorque(Ti_max_motor(1), Ti_max_motor(2), T_remaining, R(1), R(2), 1 , Mz_remaining, GR, tf);             
        end
    else
        %both false
        %Nothing to do here either
    end
end
    
Ti_all = [T_F' T_R'];

Ti_lim_struct = struct;
Ti_lim_struct.FL = Ti_all(1);
Ti_lim_struct.FR = Ti_all(2);
Ti_lim_struct.RL = Ti_all(3);
Ti_lim_struct.RR = Ti_all(4);

Ti_lim = Ti_lim_struct;
disp(Ti_lim');
% Calculate what yaw moment that was achieved with the current 
% allocation
Fx_all = prod([Ti_all; 1./R;])*GR;
Mz_allocated = L'*Fx_all';
Mz_error = Mz_ref - Mz_allocated;
end


function [T, sat] = allocateTorque(L_max, R_max, T_req,...
          R_eff_L, R_eff_R, alfa, Mz_ref, GR, t, negative_torque_limit)
      
    T = single(zeros(2,1));
    sat = uint32(0);
    % Desired torque vectoring torque
    TV_des = abs(alfa*Mz_ref*R_eff_L/(GR*t)) + abs(alfa*Mz_ref*R_eff_R/(GR*t));
    % Take absolute value since T_req can be negative in case of KERS
    T_driver = alfa*T_req;

    if ( Mz_ref <= 0)
        % Implies that left side should realize the TV torque,
        % since only torque >= 0 is used here.
        % Mz is defined positive counter clockwise
        L = min( [TV_des, T_driver, L_max]); 
        if ( (L < TV_des) ) %&& (T_driver > 0))
            % Not fulfilled desired yaw moment
            R = - min( [(TV_des - L), R_max, negative_torque_limit]);
            T = [L;R];
        else
            max_t_add = min([(L_max-TV_des), R_max, (T_driver-L)/2]);
            L = L + max_t_add;
            R = max_t_add;
            T = [L;R];
        end
        % Floats comparison
        if ( (L + 0.001) < (T_driver))
            sat = uint32(1);
        end
        return;
    else
        R = min( [TV_des, T_driver, R_max]);
        %Max torque that can be added to both  
        if ( (R < TV_des) ) % && (T_driver > 0) )
            L = -min( [(TV_des - R), L_max,negative_torque_limit]);
            T = [L;R];
        else
            max_t_add = min([(R_max - TV_des),L_max, (T_driver-R)/2]);
            R = R + max_t_add;
            L = max_t_add;
            T = [L;R];
        end
        
        if ( (R + 0.001) < (T_driver))
            sat = uint32(1);
        end
        return;
    end
end

function [T, sat] = allocateKersTorque(L_max, R_max, T_req, R_eff_L, R_eff_R, alfa, Mz_ref, GR, t )
    T = single(zeros(2,1));
    sat = uint32(0);
    % Desired torque vectoring torque
    TV_des = abs(alfa*Mz_ref*R_eff_L/(GR*t)) + abs(alfa*Mz_ref*R_eff_R/(GR*t));
    % Take absolute value since T_req can be negative in case of KERS
    T_driver = abs(alfa*T_req);
   
    if (Mz_ref + 0.0001 >= 0)
        % Positive Mz_ref requires left side (inner wheels)
        % to brake more than the outer wheels.
        L = min( [TV_des, T_driver, L_max]);
        %Max torque that can be added to both
        if L_max < abs(TV_des)
            max_t_add = single(0);
        else
            max_t_add = min([(L_max-TV_des), R_max, (T_driver-L)/2]);
        end 
        L = - (L + max_t_add);
        R = - max_t_add;
        T = [L;R];
        % Floats comparison
        if ( (abs(L) + abs(R) + 0.001) < T_driver)
            sat = uint32(1);
        end
        return;
    else
        R = min( [abs(TV_des), T_driver, R_max]);
        %Max torque that can be added to both
        if R_max < abs(TV_des)
            max_t_add = single(0);
        else
            max_t_add = min([(R_max-abs(TV_des)), L_max, (T_driver-R)/2]);
        end
        R = - (R + max_t_add);
        L = - max_t_add;
        T = [L;R];
        % Floats comparison
        if ( (abs(L) + abs(R) + 0.001) < T_driver)
            sat = uint32(1);
        end
        return;
    end
end
function [T, sat] = allocatePositiveTorque(L_max, R_max, T_req,...
          R_eff_L, R_eff_R, alfa, Mz_ref, GR, t )
      
    T = single(zeros(2,1));
    sat = uint32(0);
    % Desired torque vectoring torque
    TV_des = abs(alfa*Mz_ref*R_eff_L/(GR*t)) + abs(alfa*Mz_ref*R_eff_R/(GR*t));
    % Take absolute value since T_req can be negative in case of KERS
    T_driver = alfa*T_req;

    if ( Mz_ref <= 0)
        % Implies that left side should realize the TV torque,
        % since only torque >= 0 is used here.
        % Mz is defined positive counter clockwise
        L = min( [TV_des, T_driver, L_max]);
        %Max torque that can be added to both
        %Skal det ikke være L < TV_des
        if L_max < abs(TV_des)
            max_t_add = single(0);
        else
            max_t_add = min([(L_max-TV_des), R_max, (T_driver-L)/2]);
        end 
        L = L + max_t_add;
        R = max_t_add;
        T = [L;R];  
        % Floats comparison
        if ( (L + R + 0.001) < (T_driver))
            sat = uint32(1);
        end
        return;
    else
        R = min( [abs(TV_des), T_driver, R_max]);
        %Max torque that can be added to both
        if R_max < abs(TV_des)
            max_t_add = single(0);
        else
            max_t_add = min([(R_max-abs(TV_des)),L_max, (T_driver-R)/2]);
        end
        R = R + max_t_add;
        L = max_t_add;
        T = [L;R];
        % Floats comparison
        if ( (L + R + 0.001) < (T_driver))
            sat = uint32(1);
        end
        return;
    end
end
